simulink model "CaseStudyII_9_Bus"  (R2020a)
settings: Solver=FixedStepAuto  StartTime=0.0  StopTime=Tend  FixedStep=T_s_power  MaxStep=5.0E-5  RelTol=1e-3
values from neighbouring files (symbols this model uses):
  B_s46 = b_s46*Cb    (= 9.5071761847e-07)    [Data_CaseStudyI.m]    (also in Data_CaseStudyII.m; Data_InitialSystem.m)
  B_s54 = b_s54*Cb    (= 1.05902722057e-06)    [Data_CaseStudyI.m]    (also in Data_CaseStudyII.m; Data_InitialSystem.m)
  B_s69 = b_s69*Cb    (= 2.15415764185e-06)    [Data_CaseStudyI.m]    (also in Data_CaseStudyII.m; Data_InitialSystem.m)
  B_s75 = b_s75*Cb    (= 1.84126323577e-06)    [Data_CaseStudyI.m]    (also in Data_CaseStudyII.m; Data_InitialSystem.m)
  B_s87 = b_s87*Cb    (= 8.96562817417e-07)    [Data_CaseStudyI.m]    (also in Data_CaseStudyII.m; Data_InitialSystem.m)
  B_s98 = b_s98*Cb    (= 1.25759482443e-06)    [Data_CaseStudyI.m]    (also in Data_CaseStudyII.m; Data_InitialSystem.m)
  C_dc_DVPP_1_2 = 0.008*(n_DVPP_1_2)    (= 0.8)    [Data_CaseStudyI.m]    (also in Data_CaseStudyII.m)
  C_dc_DVPP_1_3 = 0.008*(n_DVPP_1_3)    (= 0.4)    [Data_CaseStudyI.m]    (also in Data_CaseStudyII.m)
  C_dc_DVPP_3_1 = 0.008*(n_DVPP_3_1)    (= 1.128)    [Data_CaseStudyII.m]
  C_dc_DVPP_3_2 = 0.008*(n_DVPP_3_2)    (= 0.848)    [Data_CaseStudyII.m]
  C_dc_DVPP_3_3 = 0.008*(n_DVPP_3_3)    (= 1.28)    [Data_CaseStudyII.m]
  Dp_DVPP_3_pu = 1/dp_DVPP_3    (= 33.3333333333)    [Data_CaseStudyII.m]
  Dq1_DVPP_3_pu = 100    [Data_CaseStudyII.m]
  fb = 50    [Data_CaseStudyI.m]    (also in Data_CaseStudyII.m; Data_InitialSystem.m)
  HGov_dyn = HGov_delay*H_tr_droop    [Data_CaseStudyI.m]    (also in Data_CaseStudyII.m; Data_InitialSystem.m)
  HTurb_tot = H_water_way    [Data_CaseStudyI.m]    (also in Data_CaseStudyII.m; Data_InitialSystem.m)
  I_m_DVPP_1_2 = 2/3*Sb_DVPP_1_2/V_m_DVPP_1_2    [Data_CaseStudyI.m]    (also in Data_CaseStudyII.m)
  I_m_DVPP_1_3 = 2/3*Sb_DVPP_1_3/V_m_DVPP_1_3    [Data_CaseStudyI.m]    (also in Data_CaseStudyII.m)
  I_m_DVPP_3_1 = 2/3*Sb_DVPP_3_1/V_m_DVPP_3_1    [Data_CaseStudyII.m]
  I_m_DVPP_3_2 = 2/3*Sb_DVPP_3_2/V_m_DVPP_3_2    [Data_CaseStudyII.m]
  I_m_DVPP_3_3 = 2/3*Sb_DVPP_3_3/V_m_DVPP_3_3    [Data_CaseStudyII.m]
  i_star_max = 1.3    [Data_CaseStudyI.m]    (also in Data_CaseStudyII.m)
  iabc_DVPP_1_2_0 = T0*idq0_DVPP_1_2    [Data_CaseStudyI.m]    (also in Data_CaseStudyII.m)
  iabc_DVPP_1_3_0 = T0*idq0_DVPP_1_3    [Data_CaseStudyI.m]    (also in Data_CaseStudyII.m)
  iabc_DVPP_3_1_0 = T0*idq0_DVPP_3_1    [Data_CaseStudyII.m]
  iabc_DVPP_3_2_0 = T0*idq0_DVPP_3_2    [Data_CaseStudyII.m]
  iabc_DVPP_3_3_0 = T0*idq0_DVPP_3_3    [Data_CaseStudyII.m]
  K2_DVPP_1 = [-0.0221795494247 -1.60799665656 0.160449825826 -2.94803557381 -11.8081988371 -9.75170960256 0.00463021906909 -49.1667298155]    [ControlGains_DVPP1.mat]
  K3_DVPP_1 = [-0.0591512752956 -1.61493903379 -27.2946107927 -16.2119211358 -14.3657419818 2.05688388773 -2.27328406162 0.146700393037 -150.920793597]    [ControlGains_DVPP1.mat]
  k_dc_DVPP_1_2 = eta_DVPP_1_2/(Vdc_n_DVPP_1_2*m_p_DVPP_1_2)    [Data_CaseStudyI.m]    (also in Data_CaseStudyII.m)
  k_dc_DVPP_1_3 = eta_DVPP_1_3/(Vdc_n_DVPP_1_3*m_p_DVPP_1_3)    [Data_CaseStudyI.m]    (also in Data_CaseStudyII.m)
  k_dc_DVPP_3_1 = eta_DVPP_3_1/(Vdc_n_DVPP_3_1*m_p_DVPP_3_1)    [Data_CaseStudyII.m]
  k_dc_DVPP_3_2 = eta_DVPP_3_2/(Vdc_n_DVPP_3_2*m_p_DVPP_3_2)    [Data_CaseStudyII.m]
  k_dc_DVPP_3_3 = eta_DVPP_3_3/(Vdc_n_DVPP_3_3*m_p_DVPP_3_3)    [Data_CaseStudyII.m]
  ki_i_pu = 1.19    [Data_CaseStudyI.m]    (also in Data_CaseStudyII.m)
  ki_pll = 1700    [Data_CaseStudyI.m]    (also in Data_CaseStudyII.m)
  ki_q_pu = 0.005    [Data_CaseStudyI.m]    (also in Data_CaseStudyII.m)
  kp_i_pu = 0.73    [Data_CaseStudyI.m]    (also in Data_CaseStudyII.m)
  kp_pll = 150    [Data_CaseStudyI.m]    (also in Data_CaseStudyII.m)
  kp_q_pu = 0.05    [Data_CaseStudyI.m]    (also in Data_CaseStudyII.m)
  L1_DVPP_1_2_pu = 0.0186/m_DVPP_1_2    (= 0.000372)    [Data_CaseStudyI.m]    (also in Data_CaseStudyII.m)
  L1_DVPP_1_3_pu = 0.0186/m_DVPP_1_3    (= 0.000744)    [Data_CaseStudyI.m]    (also in Data_CaseStudyII.m)
  L1_DVPP_3_1_pu = 0.0186/m_DVPP_3_1    (= 0.000263829787234)    [Data_CaseStudyII.m]
  L1_DVPP_3_2_pu = 0.0186/m_DVPP_3_2    (= 0.000350943396226)    [Data_CaseStudyII.m]
  L1_DVPP_3_3_pu = 0.0186/m_DVPP_3_3    (= 0.0002325)    [Data_CaseStudyII.m]
  l1_MVHV1 = 0    [Data_CaseStudyI.m]    (also in Data_CaseStudyII.m; Data_InitialSystem.m)
  l1_MVHV2 = 0    [Data_CaseStudyI.m]    (also in Data_CaseStudyII.m; Data_InitialSystem.m)
  l1_MVHV3 = 0    [Data_CaseStudyI.m]    (also in Data_CaseStudyII.m; Data_InitialSystem.m)
  L2_DVPP_1_2_pu = L1_DVPP_1_2_pu    (= 0.000372)    [Data_CaseStudyI.m]    (also in Data_CaseStudyII.m)
  L2_DVPP_1_3_pu = L1_DVPP_1_3_pu    (= 0.000744)    [Data_CaseStudyI.m]    (also in Data_CaseStudyII.m)
  L2_DVPP_3_1_pu = L1_DVPP_3_1_pu    (= 0.000263829787234)    [Data_CaseStudyII.m]
  L2_DVPP_3_2_pu = L1_DVPP_3_2_pu    (= 0.000350943396226)    [Data_CaseStudyII.m]
  L2_DVPP_3_3_pu = L1_DVPP_3_3_pu    (= 0.0002325)    [Data_CaseStudyII.m]
  l2_MVHV1 = l_s14    (= 0.0576)    [Data_CaseStudyI.m]    (also in Data_CaseStudyII.m; Data_InitialSystem.m)
  l2_MVHV2 = l_s72    (= 0.0625)    [Data_CaseStudyI.m]    (also in Data_CaseStudyII.m; Data_InitialSystem.m)
  l2_MVHV3 = l_s39    (= 0.0586)    [Data_CaseStudyI.m]    (also in Data_CaseStudyII.m; Data_InitialSystem.m)
  l_f_DVPP_1_2 = L_f_DVPP_1_2*w_b/Zb_DVPP_1_2    [Data_CaseStudyI.m]    (also in Data_CaseStudyII.m)
  L_f_DVPP_1_2 = (1/(n_DVPP_1_2))*600*10^-6    (= 6e-06)    [Data_CaseStudyI.m]    (also in Data_CaseStudyII.m)
  l_f_DVPP_1_3 = L_f_DVPP_1_3*w_b/Zb_DVPP_1_3    [Data_CaseStudyI.m]    (also in Data_CaseStudyII.m)
  L_f_DVPP_1_3 = (1/(n_DVPP_1_3))*600*10^-6    (= 1.2e-05)    [Data_CaseStudyI.m]    (also in Data_CaseStudyII.m)
  l_f_DVPP_3_1 = L_f_DVPP_3_1*w_b/Zb_DVPP_3_1    [Data_CaseStudyII.m]
  L_f_DVPP_3_1 = (1/(n_DVPP_3_1))*600*10^-6    (= 4.25531914894e-06)    [Data_CaseStudyII.m]
  l_f_DVPP_3_2 = L_f_DVPP_3_2*w_b/Zb_DVPP_3_2    [Data_CaseStudyII.m]
  L_f_DVPP_3_2 = (1/(n_DVPP_3_2))*600*10^-6    (= 5.66037735849e-06)    [Data_CaseStudyII.m]
  l_f_DVPP_3_3 = L_f_DVPP_3_3*w_b/Zb_DVPP_3_3    [Data_CaseStudyII.m]
  L_f_DVPP_3_3 = (1/(n_DVPP_3_3))*600*10^-6    (= 3.75e-06)    [Data_CaseStudyII.m]
  L_s46 = l_s46*Lb    (= 0.154915055408)    [Data_CaseStudyI.m]    (also in Data_CaseStudyII.m; Data_InitialSystem.m)
  L_s54 = l_s54*Lb    (= 0.143128040323)    [Data_CaseStudyI.m]    (also in Data_CaseStudyII.m; Data_InitialSystem.m)
  L_s69 = l_s69*Lb    (= 0.286256080645)    [Data_CaseStudyI.m]    (also in Data_CaseStudyII.m; Data_InitialSystem.m)
  L_s75 = l_s75*Lb    (= 0.271101346964)    [Data_CaseStudyI.m]    (also in Data_CaseStudyII.m; Data_InitialSystem.m)
  L_s87 = l_s87*Lb    (= 0.12123786945)    [Data_CaseStudyI.m]    (also in Data_CaseStudyII.m; Data_InitialSystem.m)
  L_s98 = l_s98*Lb    (= 0.16973301723)    [Data_CaseStudyI.m]    (also in Data_CaseStudyII.m; Data_InitialSystem.m)
  LPV_K1_DVPP_3 = [0.014519129833 -1.24253756746e-17 -0.00331576987938 -1.41950397655e-17 -0.00331577010739 -1.6423216922e-19 0.0145191298795 1.47256053017e-18 1.92456501739e-17 0.00968260817745 7.5102914291e-19 0.0096826081765 ... (80 elements, 8x10)]    [ControlGains_DVPP3_LPV.mat]
  LPV_K2_DVPP_3 = [0.0299413265511 -2.72480441208e-16 -0.00563144274341 -6.63344905835e-17 -0.00563144273182 -1.08918556426e-16 0.0299413268326 -1.32404731664e-16 -4.78559537004e-17 -0.00914230292149 -8.50409089014e-21 -0.00914230292147 ... (80 elements, 8x10)]    [ControlGains_DVPP3_LPV.mat]
  LPV_K3_DVPP_3 = [-0.0173301370849 5.00398589077e-17 -0.0636125194304 3.31757376688e-17 -0.0636125164794 5.41726806116e-17 -0.017330137145 2.43427565927e-17 -0.0400570975704 -5.68753124238e-17 -0.0574012283733 2.45717741258e-17 ... (192 elements, 16x12)]    [ControlGains_DVPP3_LPV.mat]
  Mp_DVPP_3_pu = 13    [Data_CaseStudyII.m]
  P_L = pL*Sb    (= 300000000)    [Data_CaseStudyI.m]    (also in Data_CaseStudyII.m; Data_InitialSystem.m)
  p_set_bus1 = P_set_bus1/SbSG1    (= 0.731707317073)    [Data_CaseStudyI.m]    (also in Data_CaseStudyII.m; Data_InitialSystem.m)
  p_set_bus2 = P_set_bus2/SbSG2    (= 0.756707317073)    [Data_CaseStudyI.m]    (also in Data_CaseStudyII.m; Data_InitialSystem.m)
  Pb_DVPP_3_1 = 37e6    (= 37000000)    [Data_CaseStudyII.m]
  Pb_DVPP_3_2 = 28e6    (= 28000000)    [Data_CaseStudyII.m]
  Pb_DVPP_3_3 = 0e6    (= 0)    [Data_CaseStudyII.m]
  pset_DVPP_1_1 = P_set_bus1/SbSG1    (= 0.731707317073)    [Data_CaseStudyI.m]    (also in Data_CaseStudyII.m)
  pset_DVPP_1_2 = 0    [Data_CaseStudyI.m]    (also in Data_CaseStudyII.m)
  pset_DVPP_1_3 = 0    [Data_CaseStudyI.m]    (also in Data_CaseStudyII.m)
  pset_DVPP_3_1 = (0.6*P_set_bus3)/Sb_DVPP_3_1    (= 0.398546964193)    [Data_CaseStudyII.m]
  pset_DVPP_3_2 = (0.4*P_set_bus3)/Sb_DVPP_3_2    (= 0.353428439945)    [Data_CaseStudyII.m]
  pset_DVPP_3_3 = 0    [Data_CaseStudyII.m]
  Q_L = qL*Sb    (= 82500000)    [Data_CaseStudyI.m]    (also in Data_CaseStudyII.m; Data_InitialSystem.m)
  qset_DVPP_1_2 = 0    [Data_CaseStudyI.m]    (also in Data_CaseStudyII.m)
  qset_DVPP_1_3 = 0    [Data_CaseStudyI.m]    (also in Data_CaseStudyII.m)
  qset_DVPP_3_1 = 0    [Data_CaseStudyII.m]
  qset_DVPP_3_2 = 0    [Data_CaseStudyII.m]
  qset_DVPP_3_3 = 0    [Data_CaseStudyII.m]
  R1_DVPP_1_2_pu = 0.00734/m_DVPP_1_2    (= 0.0001468)    [Data_CaseStudyI.m]    (also in Data_CaseStudyII.m)
  R1_DVPP_1_3_pu = 0.00734/m_DVPP_1_3    (= 0.0002936)    [Data_CaseStudyI.m]    (also in Data_CaseStudyII.m)
  R1_DVPP_3_1_pu = 0.00734/m_DVPP_3_1    (= 0.000104113475177)    [Data_CaseStudyII.m]
  R1_DVPP_3_2_pu = 0.00734/m_DVPP_3_2    (= 0.000138490566038)    [Data_CaseStudyII.m]
  R1_DVPP_3_3_pu = 0.00734/m_DVPP_3_3    (= 9.175e-05)    [Data_CaseStudyII.m]
  r1_MVHV1 = 1e-6    (= 1e-06)    [Data_CaseStudyI.m]    (also in Data_CaseStudyII.m; Data_InitialSystem.m)
  r1_MVHV2 = 1e-6    (= 1e-06)    [Data_CaseStudyI.m]    (also in Data_CaseStudyII.m; Data_InitialSystem.m)
  r1_MVHV3 = 1e-6    (= 1e-06)    [Data_CaseStudyI.m]    (also in Data_CaseStudyII.m; Data_InitialSystem.m)
  R2_DVPP_1_2_pu = R1_DVPP_1_2_pu    (= 0.0001468)    [Data_CaseStudyI.m]    (also in Data_CaseStudyII.m)
  R2_DVPP_1_3_pu = R1_DVPP_1_3_pu    (= 0.0002936)    [Data_CaseStudyI.m]    (also in Data_CaseStudyII.m)
  R2_DVPP_3_1_pu = R1_DVPP_3_1_pu    (= 0.000104113475177)    [Data_CaseStudyII.m]
  R2_DVPP_3_2_pu = R1_DVPP_3_2_pu    (= 0.000138490566038)    [Data_CaseStudyII.m]
  R2_DVPP_3_3_pu = R1_DVPP_3_3_pu    (= 9.175e-05)    [Data_CaseStudyII.m]
  r2_MVHV1 = 1e-6    (= 1e-06)    [Data_CaseStudyI.m]    (also in Data_CaseStudyII.m; Data_InitialSystem.m)
  r2_MVHV2 = 1e-6    (= 1e-06)    [Data_CaseStudyI.m]    (also in Data_CaseStudyII.m; Data_InitialSystem.m)
  r2_MVHV3 = 1e-6    (= 1e-06)    [Data_CaseStudyI.m]    (also in Data_CaseStudyII.m; Data_InitialSystem.m)
  R_dc_DVPP_1_2 = (Vdc_n_DVPP_1_2/(0.05*(Sb_DVPP_1_2)/Vdc_n_DVPP_1_2))    [Data_CaseStudyI.m]    (also in Data_CaseStudyII.m)
  R_dc_DVPP_1_3 = (Vdc_n_DVPP_1_3/(0.05*(Sb_DVPP_1_3)/Vdc_n_DVPP_1_3))    [Data_CaseStudyI.m]    (also in Data_CaseStudyII.m)
  R_dc_DVPP_3_1 = (Vdc_n_DVPP_3_1/(0.05*(Sb_DVPP_3_1)/Vdc_n_DVPP_3_1))    [Data_CaseStudyII.m]
  R_dc_DVPP_3_2 = (Vdc_n_DVPP_3_2/(0.05*(Sb_DVPP_3_2)/Vdc_n_DVPP_3_2))    [Data_CaseStudyII.m]
  R_dc_DVPP_3_3 = (Vdc_n_DVPP_3_3/(0.05*(Sb_DVPP_3_3)/Vdc_n_DVPP_3_3))    [Data_CaseStudyII.m]
  r_f_DVPP_1_2 = R_f_DVPP_1_2/Zb_DVPP_1_2    [Data_CaseStudyI.m]    (also in Data_CaseStudyII.m)
  R_f_DVPP_1_2 = 0.02/n_DVPP_1_2    (= 0.0002)    [Data_CaseStudyI.m]    (also in Data_CaseStudyII.m)
  r_f_DVPP_1_3 = R_f_DVPP_1_3/Zb_DVPP_1_3    [Data_CaseStudyI.m]    (also in Data_CaseStudyII.m)
  R_f_DVPP_1_3 = 0.02/n_DVPP_1_3    (= 0.0004)    [Data_CaseStudyI.m]    (also in Data_CaseStudyII.m)
  r_f_DVPP_3_1 = R_f_DVPP_3_1/Zb_DVPP_3_1    [Data_CaseStudyII.m]
  ... (+104 more)
undefined symbols (not defined in the file or in its folder): A, B, C, Continuous, Dd, Efd0, gcbh, i_dc, Ka, Kf, p2set, SbSM2, sps_rtmsupport, spsST1AModel, Ta, Tb, Tb1, Tc, Tc1, Tf, VA0, VAmax, VAmin, VImax, VImin, VRmax, VRmin
libraries: powerlib x95, powerlib_meascontrol x41, cstblocks x15, sps_avr x1, simulink_extras x1, simulink x1
(part 1 of 5)
settings Model: SimulationMode=accelerator  Creator=verena  LastModifiedBy=verenahaberle
settings DataIOCC: ExternalInput=getinputstruct(spec1)  FinalStateName=xFinal_c2  InitialState=xInitial_CaseStudyII  LoadInitialState=on  SaveFinalState=on  SaveOperatingPoint=on  SaveFormat=Array  ReturnWorkspaceOutputs=off  TimeSaveName=tout_c2  OutputSaveName=yout_c2  SignalLoggingName=logsout_c2  DSMLoggingName=dsmout_c2
settings OptimizationCC: BlockReduction=off
settings DebuggingCC: UnconnectedInputMsg=none  UnconnectedOutputMsg=none  UnconnectedLineMsg=none  NonCurrentReleaseOperatingPointMsg=warning

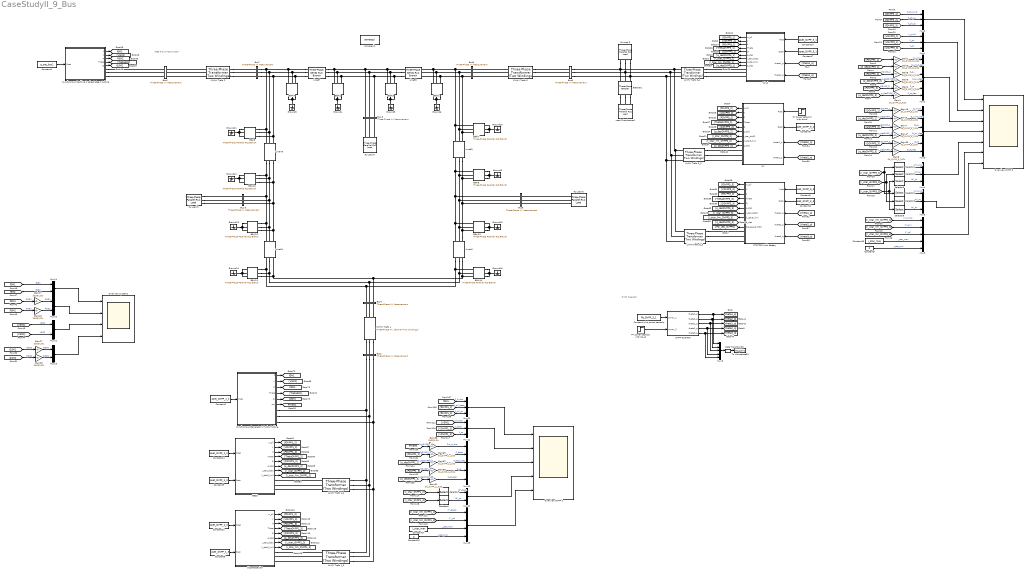
== system CaseStudyII_9_Bus ==
  note: IEEE 9-bus Test System
  note: DVPP Operator
  B94/1 : powerlib/Elements/Three-Phase Parallel RLC Branch  LConnTagsString=A|B|C  RConnTagsString=A|B|C  BranchType=C  Resistance=1  Inductance=1e-3  Capacitance=B_s98*0.5  Measurements=None
      settings: SourceProductBaseCode=PS
  B94/10 : powerlib/Elements/Three-Phase Parallel RLC Branch  LConnTagsString=A|B|C  RConnTagsString=A|B|C  BranchType=C  Resistance=1  Inductance=1e-3  Capacitance=B_s75*0.5  Measurements=None
      settings: SourceProductBaseCode=PS
  B94/11 : powerlib/Elements/Three-Phase Parallel RLC Branch  LConnTagsString=A|B|C  RConnTagsString=A|B|C  BranchType=C  Resistance=1  Inductance=1e-3  Capacitance=B_s54*0.5  Measurements=None
      settings: SourceProductBaseCode=PS
  B94/12 : powerlib/Elements/Three-Phase Parallel RLC Branch  LConnTagsString=A|B|C  RConnTagsString=A|B|C  BranchType=C  Resistance=1  Inductance=1e-3  Capacitance=B_s54*0.5  Measurements=None
      settings: SourceProductBaseCode=PS
  B94/13 : powerlib/Elements/Three-Phase Parallel RLC Branch  LConnTagsString=A|B|C  RConnTagsString=A|B|C  BranchType=C  Resistance=1  Inductance=1e-3  Capacitance=B_s46*0.5  Measurements=None
      settings: SourceProductBaseCode=PS
  B94/14 : powerlib/Elements/Three-Phase Parallel RLC Branch  LConnTagsString=A|B|C  RConnTagsString=A|B|C  BranchType=C  Resistance=1  Inductance=1e-3  Capacitance=B_s46*0.5  Measurements=None
      settings: SourceProductBaseCode=PS
  B94/2 : powerlib/Elements/Three-Phase Parallel RLC Branch  LConnTagsString=A|B|C  RConnTagsString=A|B|C  BranchType=C  Resistance=1  Inductance=1e-3  Capacitance=B_s87*0.5  Measurements=None
      settings: SourceProductBaseCode=PS
  B94/3 : powerlib/Elements/Three-Phase Parallel RLC Branch  LConnTagsString=A|B|C  RConnTagsString=A|B|C  BranchType=C  Resistance=1  Inductance=1e-3  Capacitance=B_s98*0.5  Measurements=None
      settings: SourceProductBaseCode=PS
  B94/4 : powerlib/Elements/Three-Phase Parallel RLC Branch  LConnTagsString=A|B|C  RConnTagsString=A|B|C  BranchType=C  Resistance=1  Inductance=1e-3  Capacitance=B_s87*0.5  Measurements=None
      settings: SourceProductBaseCode=PS
  B94/7 : powerlib/Elements/Three-Phase Parallel RLC Branch  LConnTagsString=A|B|C  RConnTagsString=A|B|C  BranchType=C  Resistance=1  Inductance=1e-3  Capacitance=B_s69*0.5  Measurements=None
      settings: SourceProductBaseCode=PS
  B94/8 : powerlib/Elements/Three-Phase Parallel RLC Branch  LConnTagsString=A|B|C  RConnTagsString=A|B|C  BranchType=C  Resistance=1  Inductance=1e-3  Capacitance=B_s69*0.5  Measurements=None
      settings: SourceProductBaseCode=PS
  B94/9 : powerlib/Elements/Three-Phase Parallel RLC Branch  LConnTagsString=A|B|C  RConnTagsString=A|B|C  BranchType=C  Resistance=1  Inductance=1e-3  Capacitance=B_s75*0.5  Measurements=None
      settings: SourceProductBaseCode=PS
  BESS : Subsystem
  Breaker1 : powerlib/Elements/Three-Phase Breaker  InitialState=open  SwitchA=on  SwitchB=on  SwitchC=on  SwitchTimes=[T_load_b3]  External=off  BreakerResistance=0.01  SnubberResistance=1e6  SnubberCapacitance=inf  Measurements=None
  Bus 5 : powerlib/Measurements/Three-Phase V-I Measurement  VoltageMeasurement=no  SetLabelV=on  LabelV=Vabc_5  Vpu=on  VpuLL=off  CurrentMeasurement=no  SetLabelI=on  LabelI=Iabc_5  Ipu=on  Pbase=S_b  Vbase=V_b  OutputType=Complex  PhasorSimulation=off  PSBequivalent=0
  Bus 8 : powerlib/Measurements/Three-Phase V-I Measurement  VoltageMeasurement=no  SetLabelV=on  LabelV=Vabc_9  Vpu=on  VpuLL=off  CurrentMeasurement=no  SetLabelI=on  LabelI=Iabc_9  Ipu=on  Pbase=S_b  Vbase=V_b  OutputType=Complex  PhasorSimulation=off  PSBequivalent=0
  Bus1 : powerlib/Measurements/Three-Phase V-I Measurement  VoltageMeasurement=phase-to-ground  SetLabelV=on  LabelV=Vabc_B1  Vpu=off  VpuLL=on  CurrentMeasurement=yes  SetLabelI=on  LabelI=Iabc_B1  Ipu=off  Pbase=S_b  Vbase=VbMV1  OutputType=Complex  PhasorSimulation=off  PSBequivalent=0
  Bus2 : powerlib/Measurements/Three-Phase V-I Measurement  VoltageMeasurement=no  SetLabelV=on  LabelV=Vabc_2  Vpu=off  VpuLL=off  CurrentMeasurement=no  SetLabelI=on  LabelI=Iabc_2  Ipu=on  Pbase=Sb  Vbase=VbMV2  OutputType=Complex  PhasorSimulation=off  PSBequivalent=0
  Bus3 : powerlib/Measurements/Three-Phase V-I Measurement  VoltageMeasurement=phase-to-ground  SetLabelV=on  LabelV=Vabc_B3  Vpu=off  VpuLL=on  CurrentMeasurement=yes  SetLabelI=on  LabelI=Iabc_B3  Ipu=off  Pbase=S_b  Vbase=VbMV3  OutputType=Complex  PhasorSimulation=off  PSBequivalent=0
  Bus4 : powerlib/Measurements/Three-Phase V-I Measurement  VoltageMeasurement=no  SetLabelV=off  LabelV=Vabc_6  Vpu=off  VpuLL=off  CurrentMeasurement=no  SetLabelI=off  LabelI=Iabc_6  Ipu=off  Pbase=S_b  Vbase=V_b  OutputType=Complex  PhasorSimulation=off  PSBequivalent=0
  Bus6 : powerlib/Measurements/Three-Phase V-I Measurement  VoltageMeasurement=no  SetLabelV=on  LabelV=Vabc_9  Vpu=on  VpuLL=off  CurrentMeasurement=no  SetLabelI=on  LabelI=Iabc_9  Ipu=on  Pbase=S_b  Vbase=V_b  OutputType=Complex  PhasorSimulation=off  PSBequivalent=0
  Bus7 : powerlib/Measurements/Three-Phase V-I Measurement  VoltageMeasurement=no  SetLabelV=on  LabelV=Vabc_4  Vpu=on  VpuLL=off  CurrentMeasurement=no  SetLabelI=on  LabelI=Iabc_4  Ipu=on  Pbase=S_b  Vbase=V_b  OutputType=Complex  PhasorSimulation=off  PSBequivalent=0
  Bus9 : powerlib/Measurements/Three-Phase V-I Measurement  VoltageMeasurement=phase-to-ground  SetLabelV=on  LabelV=Vabc_9  Vpu=off  VpuLL=off  CurrentMeasurement=yes  SetLabelI=on  LabelI=Iabc_9  Ipu=off  Pbase=S_b  Vbase=V_b  OutputType=Complex  PhasorSimulation=off  PSBequivalent=0
  Constant wind power capacity : Constant  Value=Pb_DVPP_3_1
  Constant1 : Constant  Value=pset_DVPP_1_1
  Constant10 : Constant  Value=pset_DVPP_3_1
  Constant11 : Constant  Value=qset_DVPP_3_3
  Constant13 : Constant  Value=i_star_max
  Constant14 : Constant  Value=qset_DVPP_1_2
  Constant17 : Constant  Value=i_star_max
  Constant18 : Constant  Value=0
  Constant21 : Constant  Value=qset_DVPP_1_3
  Constant3 : Constant  Value=0
  Constant4 : Constant  Value=p_set_bus2
  Constant5 : Constant  Value=pset_DVPP_1_2
  Constant6 : Constant  Value=pset_DVPP_1_3
  Constant7 : Constant  Value=qset_DVPP_3_1
  Constant8 : Constant  Value=qset_DVPP_3_2
  Constant9 : Constant  Value=pset_DVPP_3_3
  "DVPP Operator " : Subsystem
  Gain{1,3,9..10} (4 alike) : Gain  Gain=Sb_DVPP_3_1/Sb
  Gain17 : Gain  Gain=SbSG1/Sb
  Gain18 : Gain  Gain=SbSG2/Sb
  Gain{2,4,8,52} (4 alike) : Gain  Gain=Sb_DVPP_3_3/Sb
  Gain27 : Gain  Gain=SbSG1/Sb
  Gain28 : Gain  Gain=SbSG2/Sb
  Gain{5..7,47} (4 alike) : Gain  Gain=Sb_DVPP_3_2/Sb
  Gain58 : Gain  Gain=SbSG1/Sb
  Gain59 : Gain  Gain=Sb_DVPP_1_3/Sb
  Gain61 : Gain  Gain=Sb_DVPP_1_3/Sb
  Gain62 : Gain  Gain=Sb_DVPP_1_2/Sb
  Gain65 : Gain  Gain=Sb_DVPP_1_2/Sb
  Ground{3..6,9..16} (12 alike) : powerlib/Elements/Ground  LConnTagsString=a
  LV/MV Trafo 1_2 : powerlib/Elements/Three-Phase Transformer (Two Windings)  Winding1Connection=Yg  Winding2Connection=Yg  CoreType=Three single-phase transformers  SetSaturation=off  Hysteresis=off  DataFile='hysteresis'  SetInitialFlux=off  Measurements=None  UNITS=pu  NominalPower=[St_MVLV_DVPP_1_2, fb]  Winding1=[VbLV_DVPP_1_2,R1_DVPP_1_2_pu,L1_DVPP_1_2_pu]  Winding2=[VbMV1,R2_DVPP_1_2_pu,L2_DVPP_1_2_pu]  Rm=Rm_DVPP_1_2_pu  Lm=Lm_DVPP_1_2_pu  L0=0.5  Saturation=[ 0,0 ; 0.0024,1.2 ; 1.0,1.52 ]  InitialFluxes=[ 0.8 , -0.8 , 0.7 ]  BreakLoop=off  DiscreteSolver=Trapezoidal iterative  DataType=off  TransfoNumber=0
  LV/MV Trafo 1_3 : powerlib/Elements/Three-Phase Transformer (Two Windings)  Winding1Connection=Yg  Winding2Connection=Yg  CoreType=Three single-phase transformers  SetSaturation=off  Hysteresis=off  DataFile='hysteresis'  SetInitialFlux=off  Measurements=None  UNITS=pu  NominalPower=[St_MVLV_DVPP_1_3, fb]  Winding1=[VbLV_DVPP_1_3,R1_DVPP_1_3_pu,L1_DVPP_1_3_pu]  Winding2=[VbMV1,R2_DVPP_1_3_pu,L2_DVPP_1_3_pu]  Rm=Rm_DVPP_1_3_pu  Lm=Lm_DVPP_1_3_pu  L0=0.5  Saturation=[ 0,0 ; 0.0024,1.2 ; 1.0,1.52 ]  InitialFluxes=[ 0.8 , -0.8 , 0.7 ]  BreakLoop=off  DiscreteSolver=Trapezoidal iterative  DataType=off  TransfoNumber=0
  LV/MV Trafo 3_1 : powerlib/Elements/Three-Phase Transformer (Two Windings)  Winding1Connection=Yg  Winding2Connection=Yg  CoreType=Three single-phase transformers  SetSaturation=off  Hysteresis=off  DataFile='hysteresis'  SetInitialFlux=off  Measurements=None  UNITS=pu  NominalPower=[St_MVLV_DVPP_3_1, fb ]  Winding1=[VbLV_DVPP_3_1,R1_DVPP_3_1_pu,L1_DVPP_3_1_pu]  Winding2=[VbMV3,R2_DVPP_3_1_pu,L2_DVPP_3_1_pu]  Rm=Rm_DVPP_3_1_pu  Lm=Lm_DVPP_3_1_pu  L0=0.5  Saturation=[ 0,0 ; 0.0024,1.2 ; 1.0,1.52 ]  InitialFluxes=[0.8 -0.8 0.7]  BreakLoop=off  DiscreteSolver=Trapezoidal iterative  DataType=off  TransfoNumber=0
  LV/MV Trafo 3_2 : powerlib/Elements/Three-Phase Transformer (Two Windings)  Winding1Connection=Yg  Winding2Connection=Yg  CoreType=Three single-phase transformers  SetSaturation=off  Hysteresis=off  DataFile='hysteresis'  SetInitialFlux=off  Measurements=None  UNITS=pu  NominalPower=[St_MVLV_DVPP_3_2, fb ]  Winding1=[VbLV_DVPP_3_2,R1_DVPP_3_2_pu,L1_DVPP_3_2_pu]  Winding2=[VbMV3,R2_DVPP_3_2_pu,L2_DVPP_3_2_pu]  Rm=Rm_DVPP_3_2_pu  Lm=Lm_DVPP_3_2_pu  L0=0.5  Saturation=[ 0,0 ; 0.0024,1.2 ; 1.0,1.52 ]  InitialFluxes=[0.8 -0.8 0.7]  BreakLoop=off  DiscreteSolver=Trapezoidal iterative  DataType=off  TransfoNumber=0
  LV/MV Trafo 3_3 : powerlib/Elements/Three-Phase Transformer (Two Windings)  Winding1Connection=Yg  Winding2Connection=Yg  CoreType=Three single-phase transformers  SetSaturation=off  Hysteresis=off  DataFile='hysteresis'  SetInitialFlux=off  Measurements=None  UNITS=pu  NominalPower=[St_MVLV_DVPP_3_3, fb ]  Winding1=[VbLV_DVPP_3_3,R1_DVPP_3_3_pu,L1_DVPP_3_3_pu]  Winding2=[VbMV3,R2_DVPP_3_3_pu,L2_DVPP_3_3_pu]  Rm=Rm_DVPP_3_3_pu  Lm=Lm_DVPP_3_3_pu  L0=0.5  Saturation=[ 0,0 ; 0.0024,1.2 ; 1.0,1.52 ]  InitialFluxes=[0.8 -0.8 0.7]  BreakLoop=off  DiscreteSolver=Trapezoidal iterative  DataType=off  TransfoNumber=0
  Line46 : powerlib/Elements/Three-Phase Series RLC Branch  LConnTagsString=A|B|C  RConnTagsString=A|B|C  BranchType=RL  Resistance=R_s46  Inductance=L_s46  Capacitance=0  Measurements=None
  Line54 : powerlib/Elements/Three-Phase Series RLC Branch  LConnTagsString=A|B|C  RConnTagsString=A|B|C  BranchType=RL  Resistance=R_s54  Inductance=L_s54  Capacitance=0  Measurements=None
  Line69 : powerlib/Elements/Three-Phase Series RLC Branch  LConnTagsString=A|B|C  RConnTagsString=A|B|C  BranchType=RL  Resistance=R_s69  Inductance=L_s69  Capacitance=0  Measurements=None
  Line75 : powerlib/Elements/Three-Phase Series RLC Branch  LConnTagsString=A|B|C  RConnTagsString=A|B|C  BranchType=RL  Resistance=R_s75  Inductance=L_s75  Capacitance=0  Measurements=None
  Line87 : powerlib/Elements/Three-Phase Series RLC Branch  LConnTagsString=A|B|C  RConnTagsString=A|B|C  BranchType=RL  Resistance=R_s87  Inductance=L_s87  Capacitance=0  Measurements=None
  Line98 : powerlib/Elements/Three-Phase Series RLC Branch  LConnTagsString=A|B|C  RConnTagsString=A|B|C  BranchType=RL  Resistance=R_s98  Inductance=L_s98  Capacitance=0  Measurements=None
  Load Disturbance1 : powerlib/Elements/Three-Phase Parallel RLC Load  LConnTagsString=A|B|C  Configuration=Y (grounded)  NominalVoltage=VbMV3  Vabc=[1e3 1e3 1e3]  Vabcp=[1e3 1e3 1e3]  NominalFrequency=fb  UnbalancedPower=off  ActivePower=Load_step_b3  InductivePower=0  CapacitivePower=0  Pabc=[10e3 9e3 11e3]  QLabc=[100 90 110]  QCabc=[100 90 110]  Pabcp=[10e3 9e3 11e3]  QLabcp=[100 90 110]  QCabcp=[100 90 110]  Measurements=None  LoadType=constant Z
  "MV/HV Trafo 1 " : powerlib/Elements/Three-Phase Transformer (Two Windings)  Winding1Connection=Yg  Winding2Connection=Yg  CoreType=Three single-phase transformers  SetSaturation=off  Hysteresis=off  DataFile='hysteresis'  SetInitialFlux=off  Measurements=None  UNITS=pu  NominalPower=[St_MVHV1 fb ]  Winding1=[VbMV1 r1_MVHV1 l1_MVHV1]  Winding2=[VbHV r2_MVHV1 l2_MVHV1]  Rm=500  Lm=500  L0=0.5  Saturation="[ 0,0  ;  0.005,1.2  ;  1.0,1.4 ]"  InitialFluxes=[ 0.8 , -0.8 , 0.7 ]  BreakLoop=off  DiscreteSolver=Backward Euler robust  DataType=off  TransfoNumber=0
  "MV/HV Trafo 2 " : powerlib/Elements/Three-Phase Transformer (Two Windings)  Winding1Connection=Yg  Winding2Connection=Yg  CoreType=Three single-phase transformers  SetSaturation=off  Hysteresis=off  DataFile='hysteresis'  SetInitialFlux=off  Measurements=None  UNITS=pu  NominalPower=[St_MVHV2 fb ]  Winding1=[VbMV2 r1_MVHV2 l1_MVHV2]  Winding2=[ VbHV r2_MVHV2 l2_MVHV2]  Rm=500  Lm=500  L0=0.5  Saturation="[ 0,0  ;  0.005,1.2  ;  1.0,1.4 ]"  InitialFluxes=[ 0.8 , -0.8 , 0.7 ]  BreakLoop=off  DiscreteSolver=Backward Euler robust  DataType=off  TransfoNumber=0
  "MV/HV Trafo 3 " : powerlib/Elements/Three-Phase Transformer (Two Windings)  Winding1Connection=Yg  Winding2Connection=Yg  CoreType=Three single-phase transformers  SetSaturation=off  Hysteresis=off  DataFile='hysteresis'  SetInitialFlux=off  Measurements=None  UNITS=pu  NominalPower=[St_MVHV3 fb ]  Winding1=[VbMV3 r1_MVHV3 l1_MVHV3]  Winding2=[ VbHV r2_MVHV3 l2_MVHV3]  Rm=500  Lm=500  L0=0.5  Saturation="[ 0,0  ;  0.005,1.2  ;  1.0,1.4 ]"  InitialFluxes=[ 0.8 , -0.8 , 0.7 ]  BreakLoop=off  DiscreteSolver=Backward Euler robust  DataType=off  TransfoNumber=0
  Mux{1,4,6,8,11,21} (6 alike) : Mux  Inputs=3
  Mux{10,12..14,22} (5 alike) : Mux  Inputs=2
  Mux2 : Mux  Inputs=6
  Mux20 : Mux  Inputs=5
  Mux23 : Mux
  Mux3 : Mux  Inputs=6
  Mux5 : Mux  Inputs=5
  Mux9 : Mux  Inputs=5
  Overview DVPP 1 : Scope  NumInputPorts=5
  Overview DVPP 3 : Scope  NumInputPorts=7
  Overview System1 : Scope  NumInputPorts=4
  PV : Subsystem
  PV power capacity with cloud : Step  Time=T_cloud  Before=Pb_DVPP_3_2  After=0  SampleTime=0
  PV power setpoint with cloud : Step  Time=T_cloud  Before=pset_DVPP_3_2  After=0  SampleTime=0
  RL Load 3 : powerlib/Elements/Three-Phase Parallel RLC Load  LConnTagsString=A|B|C  Configuration=Y (grounded)  NominalVoltage=VbMV3  Vabc=[1e3 1e3 1e3]  Vabcp=[1e3 1e3 1e3]  NominalFrequency=fb  UnbalancedPower=off  ActivePower=P_L/12  InductivePower=Q_L/12  CapacitivePower=0  Pabc=[10e3 9e3 11e3]  QLabc=[100 90 110]  QCabc=[100 90 110]  Pabcp=[10e3 9e3 11e3]  QLabcp=[100 90 110]  QCabcp=[100 90 110]  Measurements=None  LoadType=constant Z
  RL Load 5 : powerlib/Elements/Three-Phase Parallel RLC Load  LConnTagsString=A|B|C  Configuration=Y (grounded)  NominalVoltage=VbHV  Vabc=[1e3 1e3 1e3]  Vabcp=[1e3 1e3 1e3]  NominalFrequency=fb  UnbalancedPower=off  ActivePower=P_L/3  InductivePower=Q_L/3  CapacitivePower=0  Pabc=[10e3 9e3 11e3]  QLabc=[100 90 110]  QCabc=[100 90 110]  Pabcp=[10e3 9e3 11e3]  QLabcp=[100 90 110]  QCabcp=[100 90 110]  Measurements=None  LoadType=constant Z
  RL Load 6 : powerlib/Elements/Three-Phase Parallel RLC Load  LConnTagsString=A|B|C  Configuration=Y (grounded)  NominalVoltage=VbHV  Vabc=[1e3 1e3 1e3]  Vabcp=[1e3 1e3 1e3]  NominalFrequency=fb  UnbalancedPower=off  ActivePower=P_L/3  InductivePower=Q_L/3  CapacitivePower=0  Pabc=[10e3 9e3 11e3]  QLabc=[100 90 110]  QCabc=[100 90 110]  Pabcp=[10e3 9e3 11e3]  QLabcp=[100 90 110]  QCabcp=[100 90 110]  Measurements=None  LoadType=constant Z
  "RL Load 8 " : powerlib/Elements/Three-Phase Parallel RLC Load  LConnTagsString=A|B|C  Configuration=Y (grounded)  NominalVoltage=VbHV  Vabc=[1e3 1e3 1e3]  Vabcp=[1e3 1e3 1e3]  NominalFrequency=fb  UnbalancedPower=off  ActivePower=P_L/4  InductivePower=Q_L/4  CapacitivePower=0  Pabc=[10e3 9e3 11e3]  QLabc=[100 90 110]  QCabc=[100 90 110]  Pabcp=[10e3 9e3 11e3]  QLabcp=[100 90 110]  QCabcp=[100 90 110]  Measurements=None  LoadType=constant Z
  Rate Transition30 : RateTransition  OutPortSampleTime=T_ms
  STATCOM with Battery : Subsystem
  Selector1 : Selector  InputPortWidth=3  IndexOptions=Index vector (dialog)  Indices=2  OutputSizes=1
  Selector{2..4,7..8} (5 alike) : Selector  InputPortWidth=3  IndexOptions=Index vector (dialog)  Indices=[1]  OutputSizes=1
  Selector5 : Selector  InputPortWidth=3  IndexOptions=Index vector (dialog)  Indices=2  OutputSizes=1
  Selector6 : Selector  InputPortWidth=3  IndexOptions=Index vector (dialog)  Indices=2  OutputSizes=1
  Supercapacitor : Subsystem
  Synchronous Generator 1 Hydro Turbine : Subsystem
  Synchronous Machine 2 reheat steam turbine : Subsystem
  To Workspace30 : ToWorkspace  VariableName=DC_gains  SampleTime=-1
  "Wind " : Subsystem
  powergui1 : powerlib/powergui  Priority=1  SimulationMode=Discrete  SampleTime=T_s_power  frequency=fb  Iterations=100  frequencyindice=0  Pbase=100e6  ErrMax=0.0001  UnitsV=kV  UnitsW=MW  buscounter=3  FunctionMessages=off  echomessages=off  EnableUseOfTLC=off  CurrentSourceSwitches=off  DisableSnubberDevices=off  DisableRonSwitches=off  DisableVfSwitches=off  DisplayEquations=off  AutomaticDiscreteSolvers=off  SolverType=Tustin/Backward Euler (TBE)  Interpol=off  ExternalGateDelay=off  methode=off  Ts=100  x0status=blocks  SPID=off  SwTol=0  HookPort=off  NonlinearTolerance=1e-5  nMaxIteration=200  ContinueOnMaxIteration=off  RestoreLinks=warning  ResistiveCurrentMeasurement=off  Frange=[0:2:500]  Ylog=off  Xlog=on  ShowGrid=off  save=off  variable=ZData  structure=0  ZoomFFT=off  StartTime=0.0  cycles=1  DisplayStyle=1  fundamental=60  FreqAxis=off  MaxFrequency=1000  frequencyindicesteady=1  RmsSteady=1  display=off
  tag scope: PSM1=global, PSM2=global, PmSM1=global, QSM1=global, QSM2=global, fSM1=global, fSM2=global
  wires:
  Constant4/1 -> Synchronous Machine 2 reheat steam turbine/1(Pset)
  Synchronous Machine 2 reheat steam turbine/1(f) -> [fSM2]
  Synchronous Machine 2 reheat steam turbine/2(V) -> [VSM2]
  Synchronous Machine 2 reheat steam turbine/3(P) -> [PSM2]
  Synchronous Machine 2 reheat steam turbine/4(Theta) -> [ThetaSM2]
  Synchronous Machine 2 reheat steam turbine/5(Q) -> [QSM2]
  Selector3/1 -> Mux4/3  "id*_st"
  [VDVPP3_2] -> Mux1/2  "V_pv"
  [q_desDVPP3_3] -> Gain8/1  "q_desDVPP_3"
  [q_desDVPP3_2] -> Gain47/1  "q_desDVPP_2"
  [fDVPP3_1] -> Mux8/1  "f_pll_wind"
  [i_star_lim_DVPP3_3] -> Mux5/3  "|i*_st|"
  [fDVPP3_3] -> Mux8/3  "f_pll_st"
  [PDVPP3_2] -> Gain6/1  "PDVPP_2"
  Selector2/1 -> Mux4/2  "id*_pv"
  [i_star_lim_DVPP3_2] -> Mux5/2  "|i*_pv|"
  [QDVPP3_2] -> Gain7/1  "QDVPP_2"
  [p_desDVPP3_2] -> Gain5/1  "p_desDVPP_2"
  [i_star_DVPP3_1] -> Selector1/1, Selector4/1
  Selector5/1 -> Mux6/2  "iq*_pv"
  Gain9/1 -> Mux3/2  "Q_wind_des"
  [i_star_DVPP3_3] -> Selector6/1, Selector3/1
  [i_star_DVPP3_2] -> Selector5/1, Selector2/1
  Constant wind power capacity/1 -> "DVPP Operator "/1(pmax_1)
  "DVPP Operator "/3(theta1_q) -> Mux9/3, [theta1_q]
  [VDVPP3_3] -> Mux1/3  "V_st"
  STATCOM with Battery/9(q_des) -> [q_desDVPP3_3]
  Gain8/1 -> Mux3/6  "Q_st_des"
  "DVPP Operator "/2(theta2_p) -> Mux9/2, [theta2_p]
  Constant8/1 -> PV/2(Qset)
  Gain7/1 -> Mux3/3  "Q_pv"
  STATCOM with Battery/8(|i_star3_lim|) -> [i_star_lim_DVPP3_3]
  "Wind "/7(i_star_dq01) -> [i_star_DVPP3_1]
  STATCOM with Battery/6(p_des) -> [p_desDVPP3_3]
  PV/4(Theta) -> [ThetaDVPP3_2]
  "Wind "/2(V) -> [VDVPP3_1]
  [theta2_p] -> PV/3(theta2_p)
  Constant10/1 -> "Wind "/1(Pset)
  [theta2_q] -> PV/4(theta2_q)
  Gain5/1 -> Mux2/4  "P_pv_des"
  [QDVPP3_1] -> Gain10/1  "QDVPP_1"
  Gain6/1 -> Mux2/3  "P_pv"
  Gain1/1 -> Mux2/1  "P_wind"
  PV/1(w_pll) -> [fDVPP3_2]
  [PDVPP3_1] -> Gain1/1
  Gain47/1 -> Mux3/4  "Q_pv_des"
  Selector1/1 -> Mux6/1  "iq*_wind"
  Gain3/1 -> Mux2/2  "P_wind_des"
  [VDVPP3_1] -> Mux1/1  "V_wind"
  Selector6/1 -> Mux6/3  "iq*_st"
  [QDVPP3_3] -> Gain52/1  "QDVPP_3"
  Gain4/1 -> Mux2/6  "P_st_des"
  [PDVPP3_3] -> Gain2/1  "PDVPP_3"
  Gain2/1 -> Mux2/5  "P_st"
  [q_desDVPP3_1] -> Gain9/1  "q_desDVPP_1"
  PV power capacity with cloud/1 -> "DVPP Operator "/2(pmax_2)
  "DVPP Operator "/4(theta2_q) -> Mux9/4, [theta2_q]
  "Wind "/6(p_des) -> [p_desDVPP3_1]
  STATCOM with Battery/3(P) -> [PDVPP3_3]
  PV/8(|i_star3_lim|) -> [i_star_lim_DVPP3_2]
  "Wind "/5(Q) -> [QDVPP3_1]
  [p_desDVPP3_1] -> Gain3/1
  "DVPP Operator "/1(theta1_p) -> [theta1_p], Mux9/1
  STATCOM with Battery/2(V) -> [VDVPP3_3]
  STATCOM with Battery/4(Theta) -> [ThetaDVPP3_3]
  PV/2(V) -> [VDVPP3_2]
  "Wind "/1(w_pll) -> [fDVPP3_1]
  PV/3(P) -> [PDVPP3_2]
  PV power setpoint with cloud/1 -> PV/1(Pset)
  "Wind "/3(P) -> [PDVPP3_1]
  [theta1_q] -> "Wind "/4(theta1_q)
  [p_desDVPP3_3] -> Gain4/1  "p_desDVPP_3"
  [theta1_p] -> "Wind "/3(theta1_p)
  Constant9/1 -> STATCOM with Battery/1(Pset)
  Gain10/1 -> Mux3/1  "Q_wind"
  [i_star_lim_DVPP3_1] -> Mux5/1  "|i*_wind|"
  "Wind "/9(q_des) -> [q_desDVPP3_1]
  Selector4/1 -> Mux4/1  "id*_wind"
  STATCOM with Battery/7(i_star_dq03) -> [i_star_DVPP3_3]
  PV/6(p_des) -> [p_desDVPP3_2]
  Constant7/1 -> "Wind "/2(Qset)
  STATCOM with Battery/1(w_pll) -> [fDVPP3_3]
  [fDVPP3_2] -> Mux8/2  "f_pll_pv"
  "Wind "/8(|i_star_lim|) -> [i_star_lim_DVPP3_1]
  PV/7(i_star_dq02) -> [i_star_DVPP3_2]
  [theta3_q] -> STATCOM with Battery/5(theta3_q)
  [theta2_p] -> STATCOM with Battery/4(theta2_p)
  [theta1_p] -> STATCOM with Battery/3(theta1_p)
  "Wind "/4(Theta) -> [ThetaDVPP3_1]
  Gain52/1 -> Mux3/5  "Q_st"
  STATCOM with Battery/5(Q) -> [QDVPP3_3]
  PV/5(Q) -> [QDVPP3_2]
  PV/9(q_des) -> [q_desDVPP3_2]
  "DVPP Operator "/5(theta3_q) -> Mux9/5, [theta3_q]
  Constant11/1 -> STATCOM with Battery/2(Qset)
  Constant18/1 -> Mux23/4  "i_star_min"
  Supercapacitor/6(p_des) -> [p_desDVPP1_3]
  Mux21/1 -> Overview DVPP 1/1
  [i_star_lim_DVPP1_3] -> Mux23/2  "|i*_sc|"
  Constant21/1 -> Supercapacitor/1(Qset)
  Mux11/1 -> Overview DVPP 1/2
  Mux22/1 -> Overview DVPP 1/4
  Mux20/1 -> Overview DVPP 1/3
  Synchronous Generator 1 Hydro Turbine/2(V) -> [VSM1]
  Constant1/1 -> Synchronous Generator 1 Hydro Turbine/1(Pset)
  Gain58/1 -> Mux20/1  "Pm_hydro"
  Supercapacitor/8(|i_star3_lim|) -> [i_star_lim_DVPP1_3]
  [PmSM1] -> Gain58/1  "PmDVPP1_1"
  Constant6/1 -> Supercapacitor/2(Pset)
  [p_desDVPP1_2] -> Gain62/1  "p_desDVPP1_2"
  Supercapacitor/2(V) -> [VDVPP1_3]
  [i_star_DVPP1_3] -> Selector8/1
  [fDVPP1_3] -> Mux21/3  "f_pll_sc"
  [p_desDVPP1_3] -> Gain61/1  "p_desDVPP1_3"
  Mux23/1 -> Overview DVPP 1/5
  [PDVPP1_2] -> Gain65/1  "PDVPP1_2"
  [i_star_DVPP1_2] -> Selector7/1
  Supercapacitor/4(Theta) -> [ThetaDVPP1_3]
  Synchronous Generator 1 Hydro Turbine/6(Pm) -> [PmSM1]
  Supercapacitor/5(Q) -> [QDVPP1_3]
  Constant17/1 -> Mux23/3  "i_star_max"
  Constant5/1 -> BESS/2(Pset)
  Supercapacitor/1(w_pll) -> [fDVPP1_3]
  Synchronous Generator 1 Hydro Turbine/4(Theta) -> [ThetaSM1]
  [VDVPP1_2] -> Mux11/2  "V_bess"
  [VDVPP1_3] -> Mux11/3  "V_sc"
  BESS/7(i_star_dq01) -> [i_star_DVPP1_2]
  BESS/3(P) -> [PDVPP1_2]
  Supercapacitor/3(P) -> [PDVPP1_3]
  BESS/6(p_des) -> [p_desDVPP1_2]
  Synchronous Generator 1 Hydro Turbine/3(P) -> [PSM1]
  [PDVPP1_3] -> Gain59/1  "PDVPP1_3"
  Supercapacitor/7(i_star_dq01) -> [i_star_DVPP1_3]
  BESS/8(|i_star3_lim|) -> [i_star_lim_DVPP1_2]
  Synchronous Generator 1 Hydro Turbine/5(Q) -> [QSM1]
  [fSM1] -> Mux21/1  "f_hydro"
  Synchronous Generator 1 Hydro Turbine/1(f) -> [fSM1]
  [fDVPP1_2] -> Mux21/2  "f_pll_bess"
  Selector7/1 -> Mux22/1  "id*_bess"
  BESS/2(V) -> [VDVPP1_2]
  BESS/1(w_pll) -> [fDVPP1_2]
  Selector8/1 -> Mux22/2  "id*_sc"
  [VSM1] -> Mux11/1  "V_hydro"
  Constant14/1 -> BESS/1(Qset)
  BESS/5(Q) -> [QDVPP1_2]
  BESS/4(Theta) -> [ThetaDVPP1_2]
  [i_star_lim_DVPP1_2] -> Mux23/1  "|i*_bess|"
  STATCOM with Battery/10(PQ_des_DVPP3) -> [PQ_des_DVPP3]
  Constant13/1 -> Mux5/4  "i_star_max"
  Constant3/1 -> Mux5/5  "i_star_min"
  Mux8/1 -> Overview DVPP 3/1
  Mux1/1 -> Overview DVPP 3/2
  Mux2/1 -> Overview DVPP 3/3
  Mux3/1 -> Overview DVPP 3/4
  Mux4/1 -> Overview DVPP 3/5
  Mux6/1 -> Overview DVPP 3/6
  Mux5/1 -> Overview DVPP 3/7
  [VSM1] -> Mux12/1  "VSG1"
  [PSM2] -> Gain18/1  "PSG2"
  [QSM1] -> Gain27/1  "QSG1"
  Mux14/1 -> Overview System1/1
  Gain28/1 -> Mux13/2  "QSG2"
  [VSM2] -> Mux12/2  "VSG2"
  [QSM2] -> Gain28/1  "QSG2"
  Mux13/1 -> Overview System1/4
  Mux12/1 -> Overview System1/3
  Gain27/1 -> Mux13/1  "QSG1"
  Gain17/1 -> Mux10/1  "PSG1"
  [fSM2] -> Mux14/2  "fSG2"
  [PSM1] -> Gain17/1  "PSG1"
  [fSM1] -> Mux14/1  "fSG1"
  Mux10/1 -> Overview System1/2
  Rate Transition30/1 -> To Workspace30/1
  Mux9/1 -> Rate Transition30/1
  Gain18/1 -> Mux10/2  "PSG2"
  Gain65/1 -> Mux20/2  "P_bess"
  Gain62/1 -> Mux20/3  "P_bess_des"
  Gain59/1 -> Mux20/4  "P_sc"
  Gain61/1 -> Mux20/5  "P_sc_des"
  connections:
  B94/1/RConn1 -- Ground6/LConn1 -- B94/1/RConn2 -- B94/1/RConn3
  B94/9/RConn1 -- Ground11/LConn1 -- B94/9/RConn3 -- B94/9/RConn2
  RL Load 6/LConn3 -- Bus6/LConn3
  Bus 5/LConn1 -- Line54/LConn1 -- B94/12/LConn1 -- Line75/RConn1 -- B94/10/LConn1
  "MV/HV Trafo 2 "/RConn1 -- Bus7/RConn1
  "MV/HV Trafo 1 "/LConn1 -- Bus1/LConn1
  B94/3/RConn3 -- B94/3/RConn1 -- B94/3/RConn2 -- Ground5/LConn1
  B94/10/LConn3 -- Line75/RConn3 -- Line54/LConn3 -- B94/12/LConn3 -- Bus 5/LConn3
  B94/13/LConn1 -- Line46/LConn1 -- Bus6/RConn1 -- B94/8/LConn1 -- Line69/RConn1
  B94/8/LConn2 -- B94/13/LConn2 -- Line46/LConn2 -- Bus6/RConn2 -- Line69/RConn2
  Ground16/LConn1 -- B94/14/RConn3 -- B94/14/RConn1 -- B94/14/RConn2
  B94/11/RConn2 -- Ground14/LConn1 -- B94/11/RConn3 -- B94/11/RConn1
  Line87/LConn2 -- B94/4/LConn2 -- Bus7/LConn2 -- Line75/LConn2 -- B94/9/LConn2
  B94/2/RConn1 -- Ground4/LConn1 -- B94/2/RConn2 -- B94/2/RConn3
  "MV/HV Trafo 3 "/LConn1 -- Bus3/LConn1
  Line98/LConn2 -- B94/3/LConn2 -- Bus 8/RConn2 -- B94/2/LConn2 -- Line87/RConn2
  Line98/RConn2 -- B94/1/LConn2 -- B94/7/LConn2 -- Line69/LConn2 -- Bus9/RConn2
  Line98/LConn3 -- B94/3/LConn3 -- Bus 8/RConn1 -- Line87/RConn3 -- B94/2/LConn3
  RL Load 6/LConn1 -- Bus6/LConn1
  B94/11/LConn2 -- Line54/RConn2 -- Line46/RConn2 -- B94/14/LConn2 -- Bus4/LConn2
  Ground12/LConn1 -- B94/10/RConn3 -- B94/10/RConn1 -- B94/10/RConn2
  B94/14/LConn3 -- Line46/RConn3 -- Bus4/LConn3 -- B94/11/LConn3 -- Line54/RConn3
  Line54/RConn1 -- B94/11/LConn1 -- Bus4/LConn1 -- Line46/RConn1 -- B94/14/LConn1
  "MV/HV Trafo 3 "/RConn1 -- Bus9/LConn1
  B94/2/LConn1 -- Line87/RConn1 -- Bus 8/RConn3 -- B94/3/LConn1 -- Line98/LConn1
  Line98/RConn3 -- B94/1/LConn3 -- Bus9/RConn3 -- B94/7/LConn3 -- Line69/LConn3
  Line87/LConn3 -- B94/4/LConn3 -- Bus7/LConn3 -- B94/9/LConn3 -- Line75/LConn3
  Line46/LConn3 -- B94/8/LConn3 -- Line69/RConn3 -- Bus6/RConn3 -- B94/13/LConn3
  "MV/HV Trafo 2 "/LConn1 -- Bus2/LConn1
  B94/8/RConn3 -- B94/8/RConn1 -- B94/8/RConn2 -- Ground9/LConn1
  Line98/RConn1 -- B94/1/LConn1 -- Bus9/RConn1 -- B94/7/LConn1 -- Line69/LConn1
  B94/10/LConn2 -- Line75/RConn2 -- Line54/LConn2 -- B94/12/LConn2 -- Bus 5/LConn2
  B94/4/RConn3 -- B94/4/RConn1 -- B94/4/RConn2 -- Ground3/LConn1
  Line87/LConn1 -- B94/4/LConn1 -- B94/9/LConn1 -- Line75/LConn1 -- Bus7/LConn1
  B94/7/RConn1 -- Ground10/LConn1 -- B94/7/RConn3 -- B94/7/RConn2
  B94/12/RConn1 -- Ground13/LConn1 -- B94/12/RConn3 -- B94/12/RConn2
  RL Load 6/LConn2 -- Bus6/LConn2
  B94/13/RConn1 -- Ground15/LConn1 -- B94/13/RConn3 -- B94/13/RConn2
  Synchronous Machine 2 reheat steam turbine/RConn3 -- Bus2/RConn3
  "RL Load 8 "/LConn3 -- Bus 8/LConn1
  "MV/HV Trafo 3 "/LConn2 -- Bus3/LConn2
  "MV/HV Trafo 3 "/RConn2 -- Bus9/LConn2
  "MV/HV Trafo 1 "/LConn3 -- Bus1/LConn3
  "MV/HV Trafo 1 "/RConn1 -- Bus4/RConn1
  "MV/HV Trafo 2 "/RConn3 -- Bus7/RConn3
  RL Load 5/LConn2 -- Bus 5/RConn2
  "MV/HV Trafo 2 "/RConn2 -- Bus7/RConn2
  "MV/HV Trafo 1 "/RConn2 -- Bus4/RConn2
  "RL Load 8 "/LConn2 -- Bus 8/LConn2
  "MV/HV Trafo 2 "/LConn2 -- Bus2/LConn2
  RL Load 5/LConn3 -- Bus 5/RConn3
  "RL Load 8 "/LConn1 -- Bus 8/LConn3
  Synchronous Machine 2 reheat steam turbine/RConn1 -- Bus2/RConn1
  "MV/HV Trafo 2 "/LConn3 -- Bus2/LConn3
  "MV/HV Trafo 1 "/LConn2 -- Bus1/LConn2
  "MV/HV Trafo 3 "/RConn3 -- Bus9/LConn3
  RL Load 5/LConn1 -- Bus 5/RConn1
  Synchronous Machine 2 reheat steam turbine/RConn2 -- Bus2/RConn2
  "MV/HV Trafo 1 "/RConn3 -- Bus4/RConn3
  Bus3/LConn3 -- "MV/HV Trafo 3 "/LConn3
  LV/MV Trafo 3_1/RConn3 -- LV/MV Trafo 3_3/RConn3 -- LV/MV Trafo 3_2/RConn3 -- Breaker1/RConn3 -- Bus3/RConn3 -- RL Load 3/LConn3
  LV/MV Trafo 1_3/RConn2 -- Bus1/RConn2 -- Synchronous Generator 1 Hydro Turbine/RConn2 -- LV/MV Trafo 1_2/RConn2
  LV/MV Trafo 1_3/RConn3 -- LV/MV Trafo 1_2/RConn3 -- Bus1/RConn3 -- Synchronous Generator 1 Hydro Turbine/RConn3
  LV/MV Trafo 1_3/RConn1 -- Bus1/RConn1 -- Synchronous Generator 1 Hydro Turbine/RConn1 -- LV/MV Trafo 1_2/RConn1
  LV/MV Trafo 1_2/LConn1 -- BESS/RConn1
  LV/MV Trafo 1_2/LConn3 -- BESS/RConn3
  Supercapacitor/RConn1 -- LV/MV Trafo 1_3/LConn1
  LV/MV Trafo 1_3/LConn2 -- Supercapacitor/RConn2
  LV/MV Trafo 1_2/LConn2 -- BESS/RConn2
  LV/MV Trafo 1_3/LConn3 -- Supercapacitor/RConn3
  LV/MV Trafo 3_1/LConn1 -- "Wind "/RConn1
  LV/MV Trafo 3_1/LConn2 -- "Wind "/RConn2
  LV/MV Trafo 3_1/LConn3 -- "Wind "/RConn3
  LV/MV Trafo 3_3/LConn3 -- STATCOM with Battery/RConn3
  LV/MV Trafo 3_3/LConn2 -- STATCOM with Battery/RConn2
  LV/MV Trafo 3_3/LConn1 -- STATCOM with Battery/RConn1
  LV/MV Trafo 3_2/LConn3 -- PV/RConn3
  LV/MV Trafo 3_2/LConn2 -- PV/RConn2
  LV/MV Trafo 3_2/LConn1 -- PV/RConn1
  Breaker1/LConn1 -- Load Disturbance1/LConn1
  Breaker1/LConn3 -- Load Disturbance1/LConn3
  Breaker1/LConn2 -- Load Disturbance1/LConn2
  LV/MV Trafo 3_2/RConn2 -- LV/MV Trafo 3_1/RConn2 -- Breaker1/RConn2 -- RL Load 3/LConn2 -- Bus3/RConn2 -- LV/MV Trafo 3_3/RConn2
  LV/MV Trafo 3_3/RConn1 -- LV/MV Trafo 3_1/RConn1 -- Breaker1/RConn1 -- Bus3/RConn1 -- RL Load 3/LConn1 -- LV/MV Trafo 3_2/RConn1
